simulink model "Hardware_Model"  (R2022b)
settings: Solver=ode5  StartTime=0.0  StopTime=365  RelTol=1e-3  EnableMultiTasking=on
undefined symbols (not defined in the file or in its folder): cf, conv, sf, uc, vf
libraries: arduinolib x9, simulink x5, dspsigops x1
settings Model: SimulationMode=external  ExtModeTrigDuration=2  Creator=gotta  LastModifiedBy=gotta
settings SolverCC: AutoInsertRateTranBlk=on
settings OptimizationCC: EnhancedBackFolding=on  PassReuseOutputArgsAs=Individual arguments  ZeroExternalMemoryAtStartup=off  ZeroInternalMemoryAtStartup=off  MaxStackSize=64  OptimizeBlockOrder=speed  DifferentSizesBufferReuse=on  OptimizationCustomize=off  EfficientTunableParamExpr=on
settings DebuggingCC: ParameterTunabilityLossMsg=error
settings HardwareCC: ProdBitPerPointer=32  ProdBitPerSizeT=32  ProdBitPerPtrDiffT=32  ProdLargestAtomicInteger=Long  ProdLargestAtomicFloat=Double  ProdWordSize=32  ProdHWDeviceType=ARM Compatible->ARM Cortex
settings SFSimCC: MATLABDynamicMemAlloc=off
settings RTWCC: Description=Embedded Coder  SystemTargetFile=ert.tlc  HardwareBoard=ESP32-WROOM(Arduino Compatible)  TemplateMakefile=ert_default_tmf  Toolchain=ESP32  BuildConfiguration=Faster Runs
settings CodeAppCC: ForceParamTrailComments=on  IgnoreCustomStorageClasses=off  OperatorAnnotations=on  SimulinkDataObjDesc=on  SFDataObjDesc=on  InsertBlockDesc=on
settings ERTTargetCC: SupportContinuousTime=on  SupportVariableSizeSignals=on  ExtMode=on  ExtModeTransport=3  ExtModeStaticAlloc=on  ExtModeAutomaticAllocSize=off  ExtModeStaticAllocSize=65536  ExtModeMexFile=ext_xcp  ExtModeMexArgs=0 3 921600  ExtModeIntrfLevel=Level2 - Open

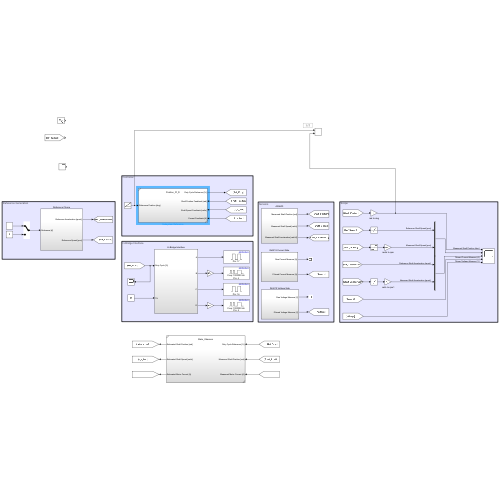
[thumbnail: Simulink's stored preview of the top-level diagram]
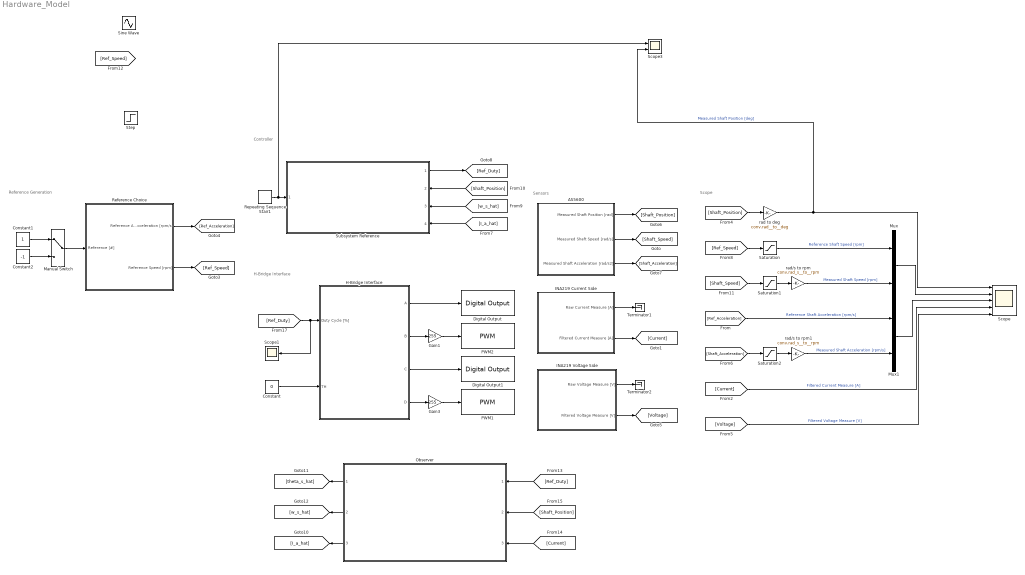
== system Hardware_Model ==
  note: Scope
  note: Sensors
  note: Controller
  note: H-Bridge Interface
  note: Reference Generation
  AS5600 : Subsystem
  Constant : Constant  Value=0
  Constant1 : Constant
  Constant2 : Constant  Value=-1
  Digital Output : arduinolib/Digital Output  pinNumber=17  Direction=output  blockPlatform=arduino
  Digital Output1 : arduinolib/Digital Output  pinNumber=16  Direction=output  blockPlatform=arduino
  Gain1 : Gain  Gain=255
  Gain3 : Gain  Gain=255
  H-Bridge Interface : Subsystem
  INA219 Current Side : Subsystem
  INA219 Voltage Side : Subsystem
  Manual Switch : ManualSwitch
  Mux : Mux  Inputs=2
  Mux1 : Mux  Inputs=2
  Observer : Subsystem  ReferencedSubsystem=State_Observer
  PWM1 : arduinolib/PWM  pinNumber=5  frequencyType=Specify  desiredFrequency=1e6  achievableFrequency=1000000
  PWM2 : arduinolib/PWM  pinNumber=4  frequencyType=Specify  desiredFrequency=1e6  achievableFrequency=1000000
  Reference Choice : Subsystem
  Repeating Sequence Stair1 : simulink/Sources/Repeating Sequence Stair  OutValues=5*[0:1:72]  tsamp=5  OutMin=[]  OutMax=[]  OutDataTypeStr=double  OutputDataTypeScalingMode=double  OutDataType=fixdt(0,8)  ConRadixGroup=Best Precision: Vector-wise  OutScaling=2^-12
  Saturation : Saturate  UpperLimit=130  LowerLimit=-130
  Saturation1 : Saturate  UpperLimit=130  LowerLimit=-130
  Saturation2 : Saturate  UpperLimit=50  LowerLimit=-50
  Scope : Scope  NumInputPorts=5
  Scope1 : Scope
  Scope3 : Scope  NumInputPorts=2
  Sine Wave : Sin  Amplitude=90  SampleTime=0
  Step : Step  After=100  SampleTime=0
  Subsystem Reference : Subsystem  ReferencedSubsystem=Position_PI_D
      settings: PortSchema="{\"entries\":[{\"content\":{\"sides\":[{\"content\":{\"connectorIds\":[\"In1\"]},\"type\":\"ConnectorPlacement.EquallySpacedRectSide\",\"uuid\":\"89c992bc-e0f3-428d-980e-b961eb5d7b7b\"},{\"content\":{\"connectorIds\":[\"Out1\",\"In2\",\"In3\",\"In4\"],\"side\":\"RIGHT\"},\"type\":\"ConnectorPlacement.EquallySpacedRectSide\",\"uuid\":\"dbaab0ea-2322-47c9-b2e4-ea83bc14c20f\"},{\"content\":{\"connectorIds\":[],\"side\":\"TOP\"},\"type\":\"ConnectorPlacement.EquallySpacedRectSide\",\"uuid\":\"a9d5f6a0-5f2c-4e6a-b514-fb4908ab5e4d\"}]},\"type\":\"ConnectorPlacement.EquallySpacedConnector\",\"uuid\":\"ac98b5ea-1932-4944-bc3f-916f19a2da62\"}],\"packageUris\":[\"http://schema.mathworks.com/mf0/Connector/R2020b\"],\"version\":\"1.0\"}"
  Terminator1 : Terminator
  Terminator2 : Terminator
  rad to deg : Gain  Gain=conv.rad__to__deg
  rad/s to rpm : Gain  Gain=conv.rad_s__to__rpm
  rad/s to rpm1 : Gain  Gain=conv.rad_s__to__rpm
  wires:
  Manual Switch/1 -> Reference Choice/1(Reference [#])
  Constant1/1 -> Manual Switch/1
  Constant2/1 -> Manual Switch/2
  Reference Choice/1(Reference Acceleration [rpm/s]) -> [Ref_Acceleration]
  Reference Choice/2(Reference Speed [rpm]) -> [Ref_Speed]
  H-Bridge Interface/4(D) -> Gain3/1
  H-Bridge Interface/2(B) -> Gain1/1
  H-Bridge Interface/3(C) -> Digital Output1/1
  [Ref_Duty] -> Scope1/1, H-Bridge Interface/1(Duty Cycle [%])
  Constant/1 -> H-Bridge Interface/2(TH)
  H-Bridge Interface/1(A) -> Digital Output/1
  Gain1/1 -> PWM2/1
  Gain3/1 -> PWM1/1
  INA219 Current Side/2(Filtered Current Measure [A]) -> [Current]
  AS5600/2(Measured Shaft Speed [rad/s]) -> [Shaft_Speed]
  INA219 Voltage Side/2(Filtered Voltage Measure [V]) -> [Voltage]
  AS5600/3(Measured Shaft Acceleration [rad/s2]) -> [Shaft_Acceleration]
  AS5600/1(Measured Shaft Position [rad]) -> [Shaft_Position]
  [Current] -> Scope/4  "Filtered Current Measure [A]"
  Saturation1/1 -> rad/s to rpm/1
  Saturation/1 -> Mux/1  "Reference Shaft Speed [rpm]"
  [Shaft_Acceleration] -> Saturation2/1
  Mux/1 -> Scope/2
  rad/s to rpm1/1 -> Mux1/2  "Measured Shaft Acceleration [rpm/s]"
  [Ref_Acceleration] -> Mux1/1  "Reference Shaft Acceleration [rpm/s]"
  rad/s to rpm/1 -> Mux/2  "Measured Shaft Speed [rpm]"
  [Shaft_Speed] -> Saturation1/1
  [Ref_Speed] -> Saturation/1
  [Voltage] -> Scope/5  "Filtered Voltage Measure [V]"
  [Shaft_Position] -> rad to deg/1
  Mux1/1 -> Scope/3
  rad to deg/1 -> Scope3/2, Scope/1  "Measured Shaft Position [deg]"
  Saturation2/1 -> rad/s to rpm1/1
  INA219 Current Side/1(Raw Current Measure [A]) -> Terminator1/1
  INA219 Voltage Side/1(Raw Voltage Measure [V]) -> Terminator2/1
  [I_a_hat] -> Subsystem Reference/4
  [w_s_hat] -> Subsystem Reference/3
  [Shaft_Position] -> Subsystem Reference/2
  Observer/1 -> [theta_s_hat]
  Observer/3 -> [I_a_hat]
  Observer/2 -> [w_s_hat]
  [Ref_Duty] -> Observer/1
  [Current] -> Observer/3
  [Shaft_Position] -> Observer/2
  Subsystem Reference/1 -> [Ref_Duty]
  Repeating Sequence Stair1/1 -> Scope3/1, Subsystem Reference/1

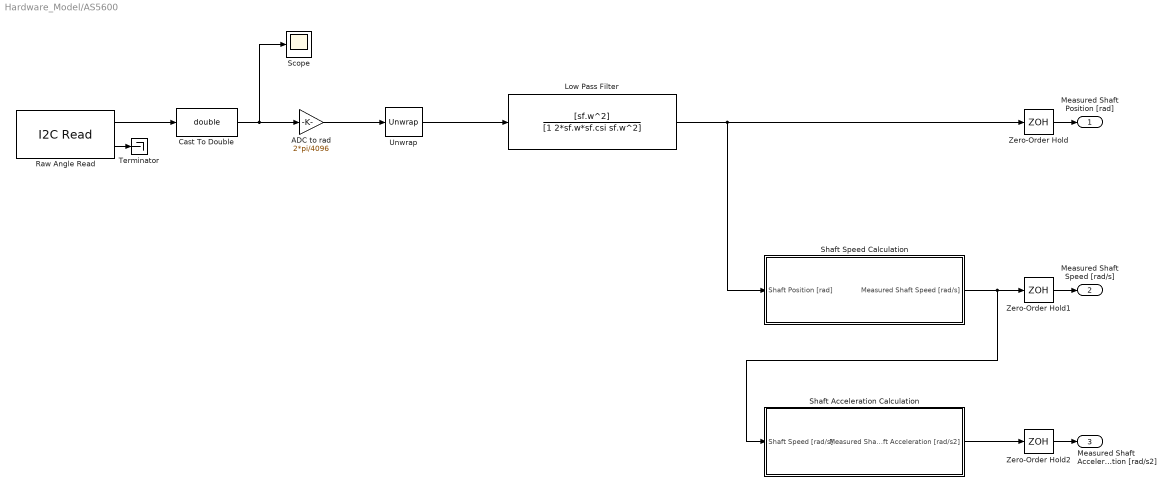
== system Hardware_Model/AS5600 ==
  ADC to rad : Gain  Gain=2*pi/4096
  Cast To Double : DataTypeConversion  OutDataTypeStr=double  SaturateOnIntegerOverflow=off  RndMeth=Floor
  Low Pass Filter : TransferFcn  Numerator=[sf.w^2]  Denominator=[1 2*sf.w*sf.csi sf.w^2]
  Raw Angle Read : arduinolib/I2C Read  I2CModule=0  Mode=Master  SlaveAddress=0x36  SlaveByteOrder=BigEndian  Direction=Receiver  RegisterAddressMode=on  RegisterAddress=0x0C  SlaveDataType=uint16  DataLength=1  NoAck=off  RepeatedStart=off  OutputStatus=on  blockPlatform=ARDUINO  SampleTime=uc.Ts
  Scope : Scope
  Shaft Acceleration Calculation : Subsystem
  Shaft Speed Calculation : Subsystem
  Terminator : Terminator
  Unwrap : dspsigops/Unwrap  tol=pi  InputProcessing=Columns as channels (frame based)  running=off
  Zero-Order Hold : ZeroOrderHold  SampleTime=uc.Ts
  Zero-Order Hold1 : ZeroOrderHold  SampleTime=uc.Ts
  Zero-Order Hold2 : ZeroOrderHold  SampleTime=uc.Ts
  Measured Shaft Position [rad] : Outport
  Measured Shaft Speed [rad/s] : Outport  Port=2
  Measured Shaft Acceleration [rad/s2] : Outport  Port=3
  wires:
  ADC to rad/1 -> Unwrap/1
  Cast To Double/1 -> Scope/1, ADC to rad/1
  Raw Angle Read/1 -> Cast To Double/1
  Unwrap/1 -> Low Pass Filter/1
  Raw Angle Read/2 -> Terminator/1
  Shaft Speed Calculation/1(Measured Shaft Speed [rad/s]) -> Shaft Acceleration Calculation/1(Shaft Speed [rad/s]), Zero-Order Hold1/1
  Shaft Acceleration Calculation/1(Measured Shaft Acceleration [rad/s2]) -> Zero-Order Hold2/1
  Low Pass Filter/1 -> Shaft Speed Calculation/1(Shaft Position [rad]), Zero-Order Hold/1
  Zero-Order Hold/1 -> Measured Shaft Position [rad]/1
  Zero-Order Hold1/1 -> Measured Shaft Speed [rad/s]/1
  Zero-Order Hold2/1 -> Measured Shaft Acceleration [rad/s2]/1

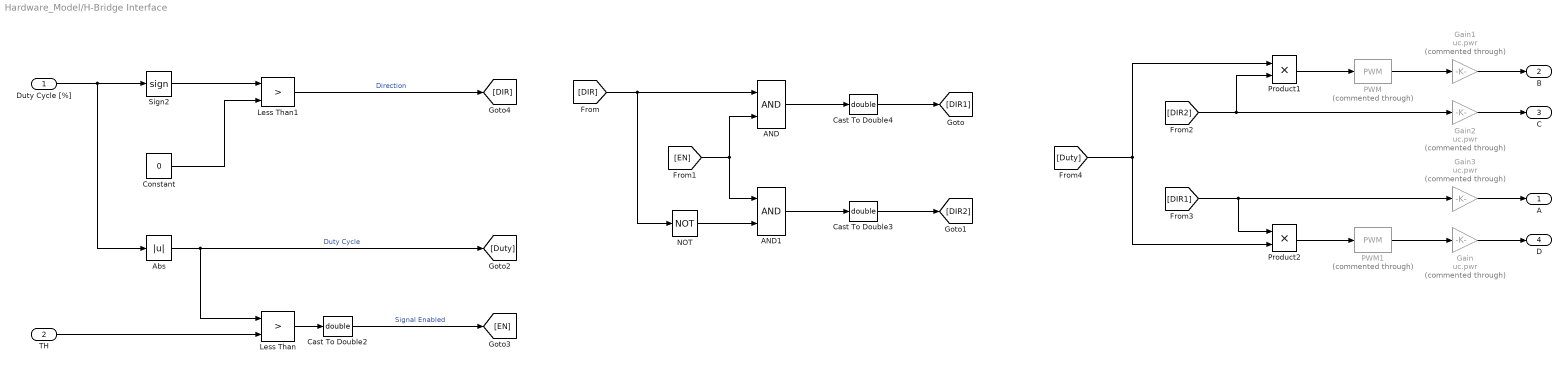
== system Hardware_Model/H-Bridge Interface ==
  Duty Cycle [%] : Inport
  TH : Inport  Port=2
  AND : Logic  IconShape=distinctive  AllPortsSameDT=off  OutDataTypeStr=boolean
  AND1 : Logic  IconShape=distinctive  AllPortsSameDT=off  OutDataTypeStr=boolean
  Abs : Abs  SaturateOnIntegerOverflow=off
  Cast To Double2 : DataTypeConversion  OutDataTypeStr=double  SaturateOnIntegerOverflow=off  RndMeth=Floor
  Cast To Double3 : DataTypeConversion  OutDataTypeStr=double  SaturateOnIntegerOverflow=off  RndMeth=Floor
  Cast To Double4 : DataTypeConversion  OutDataTypeStr=double  SaturateOnIntegerOverflow=off  RndMeth=Floor
  Constant : Constant  Value=0
  Gain{,1..3} (4 alike) : Gain  Commented=through  Gain=uc.pwr
  Less Than : RelationalOperator  Operator=>  OutDataTypeStr=boolean  RndMeth=Simplest  InputSameDT=off
  Less Than1 : RelationalOperator  Operator=>  OutDataTypeStr=boolean  RndMeth=Simplest  InputSameDT=off
  NOT : Logic  Operator=NOT  IconShape=distinctive  AllPortsSameDT=off  OutDataTypeStr=boolean
  PWM : simulink/Discontinuities/PWM  Commented=through  DisableCoverage=on  Period=uc.Tpwm  InitialDelay=0  DisallowZeroDutyCycle=off  RunAtFixedTimeIntervals=on  SampleTime=uc.Tpwm/10
  PWM1 : simulink/Discontinuities/PWM  Commented=through  DisableCoverage=on  Period=uc.Tpwm  InitialDelay=0  DisallowZeroDutyCycle=off  RunAtFixedTimeIntervals=on  SampleTime=uc.Tpwm/10
  Product1 : Product
  Product2 : Product
  Sign2 : Signum
  A : Outport
  B : Outport  Port=2
  C : Outport  Port=3
  D : Outport  Port=4
  wires:
  TH/1 -> Less Than/2
  Duty Cycle [%]/1 -> Abs/1, Sign2/1
  Less Than/1 -> Cast To Double2/1
  Sign2/1 -> Less Than1/1
  Constant/1 -> Less Than1/2
  Abs/1 -> [Duty], Less Than/1  "Duty Cycle"
  Gain/1 -> D/1
  Gain1/1 -> B/1
  Gain2/1 -> C/1
  Gain3/1 -> A/1
  AND1/1 -> Cast To Double3/1
  AND/1 -> Cast To Double4/1
  NOT/1 -> AND1/2
  Product1/1 -> PWM/1
  Product2/1 -> PWM1/1
  Cast To Double2/1 -> [EN]  "Signal Enabled"
  Less Than1/1 -> [DIR]  "Direction"
  [DIR] -> NOT/1, AND/1
  [EN] -> AND/2, AND1/1
  Cast To Double4/1 -> [DIR1]
  Cast To Double3/1 -> [DIR2]
  [DIR2] -> Product1/2, Gain2/1
  [DIR1] -> Product2/1, Gain3/1
  [Duty] -> Product1/1, Product2/2
  PWM/1 -> Gain1/1
  PWM1/1 -> Gain/1

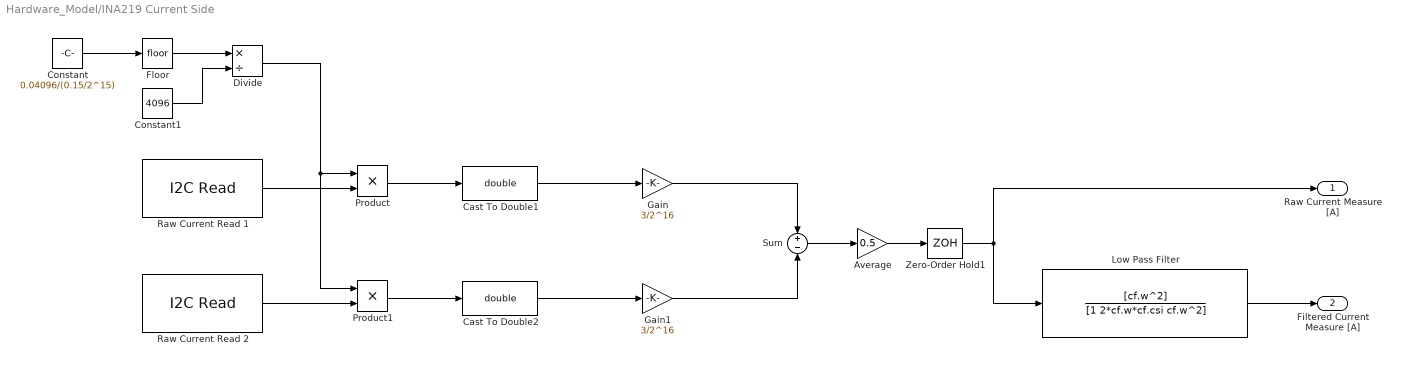
== system Hardware_Model/INA219 Current Side ==
  Average : Gain  Gain=0.5
  Cast To Double1 : DataTypeConversion  OutDataTypeStr=double  SaturateOnIntegerOverflow=off  RndMeth=Floor
  Cast To Double2 : DataTypeConversion  OutDataTypeStr=double  SaturateOnIntegerOverflow=off  RndMeth=Floor
  Constant : Constant  Value=0.04096/(0.15/2^15)
  Constant1 : Constant  Value=4096
  Divide : Product  Inputs=*/
  Floor : Rounding
  Gain : Gain  Gain=3/2^16
  Gain1 : Gain  Gain=3/2^16
  Low Pass Filter : TransferFcn  Numerator=[cf.w^2]  Denominator=[1 2*cf.w*cf.csi cf.w^2]
  Product : Product
  Product1 : Product
  Raw Current Read 1 : arduinolib/I2C Read  I2CModule=0  Mode=Master  SlaveAddress=0x40  SlaveByteOrder=BigEndian  Direction=Receiver  RegisterAddressMode=on  RegisterAddress=0x01  SlaveDataType=int16  DataLength=1  NoAck=off  RepeatedStart=off  OutputStatus=off  blockPlatform=ARDUINO  SampleTime=uc.Ts
  Raw Current Read 2 : arduinolib/I2C Read  I2CModule=0  Mode=Master  SlaveAddress=0x44  SlaveByteOrder=BigEndian  Direction=Receiver  RegisterAddressMode=on  RegisterAddress=0x01  SlaveDataType=int16  DataLength=1  NoAck=off  RepeatedStart=off  OutputStatus=off  blockPlatform=ARDUINO  SampleTime=uc.Ts
  Sum : Sum  Inputs=+|-
  Zero-Order Hold1 : ZeroOrderHold  SampleTime=uc.Ts
  Raw Current Measure [A] : Outport
  Filtered Current Measure [A] : Outport  Port=2
  wires:
  Average/1 -> Zero-Order Hold1/1
  Sum/1 -> Average/1
  Low Pass Filter/1 -> Filtered Current Measure [A]/1
  Constant/1 -> Floor/1
  Floor/1 -> Divide/1
  Constant1/1 -> Divide/2
  Raw Current Read 2/1 -> Product1/2
  Raw Current Read 1/1 -> Product/2
  Divide/1 -> Product1/1, Product/1
  Product/1 -> Cast To Double1/1
  Product1/1 -> Cast To Double2/1
  Gain/1 -> Sum/1
  Gain1/1 -> Sum/2
  Cast To Double1/1 -> Gain/1
  Cast To Double2/1 -> Gain1/1
  Zero-Order Hold1/1 -> Low Pass Filter/1, Raw Current Measure [A]/1

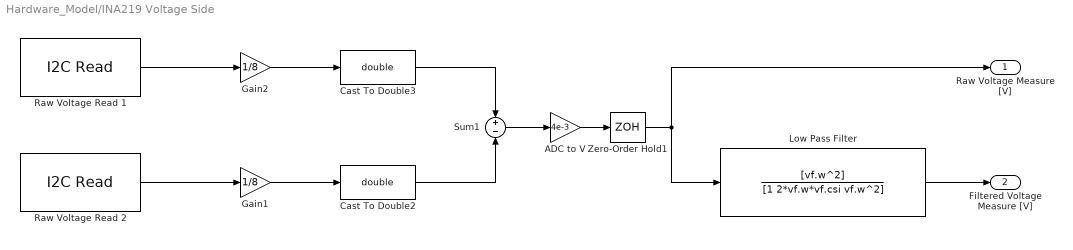
== system Hardware_Model/INA219 Voltage Side ==
  ADC to V : Gain  Gain=4e-3
  Cast To Double2 : DataTypeConversion  OutDataTypeStr=double  SaturateOnIntegerOverflow=off  RndMeth=Floor
  Cast To Double3 : DataTypeConversion  OutDataTypeStr=double  SaturateOnIntegerOverflow=off  RndMeth=Floor
  Gain1 : Gain  Gain=1/8
  Gain2 : Gain  Gain=1/8
  Low Pass Filter : TransferFcn  Numerator=[vf.w^2]  Denominator=[1 2*vf.w*vf.csi vf.w^2]
  Raw Voltage Read 1 : arduinolib/I2C Read  I2CModule=0  Mode=Master  SlaveAddress=0x40  SlaveByteOrder=BigEndian  Direction=Receiver  RegisterAddressMode=on  RegisterAddress=0x02  SlaveDataType=uint16  DataLength=1  NoAck=off  RepeatedStart=off  OutputStatus=off  blockPlatform=ARDUINO  SampleTime=uc.Ts
  Raw Voltage Read 2 : arduinolib/I2C Read  I2CModule=0  Mode=Master  SlaveAddress=0x44  SlaveByteOrder=BigEndian  Direction=Receiver  RegisterAddressMode=on  RegisterAddress=0x02  SlaveDataType=uint16  DataLength=1  NoAck=off  RepeatedStart=off  OutputStatus=off  blockPlatform=ARDUINO  SampleTime=uc.Ts
  Sum1 : Sum  Inputs=+|-
  Zero-Order Hold1 : ZeroOrderHold  SampleTime=uc.Ts
  Raw Voltage Measure [V] : Outport
  Filtered Voltage Measure [V] : Outport  Port=2
  wires:
  Cast To Double2/1 -> Sum1/2
  Gain1/1 -> Cast To Double2/1
  Raw Voltage Read 1/1 -> Gain2/1
  Sum1/1 -> ADC to V/1
  Raw Voltage Read 2/1 -> Gain1/1
  Gain2/1 -> Cast To Double3/1
  Cast To Double3/1 -> Sum1/1
  ADC to V/1 -> Zero-Order Hold1/1
  Low Pass Filter/1 -> Filtered Voltage Measure [V]/1
  Zero-Order Hold1/1 -> Low Pass Filter/1, Raw Voltage Measure [V]/1

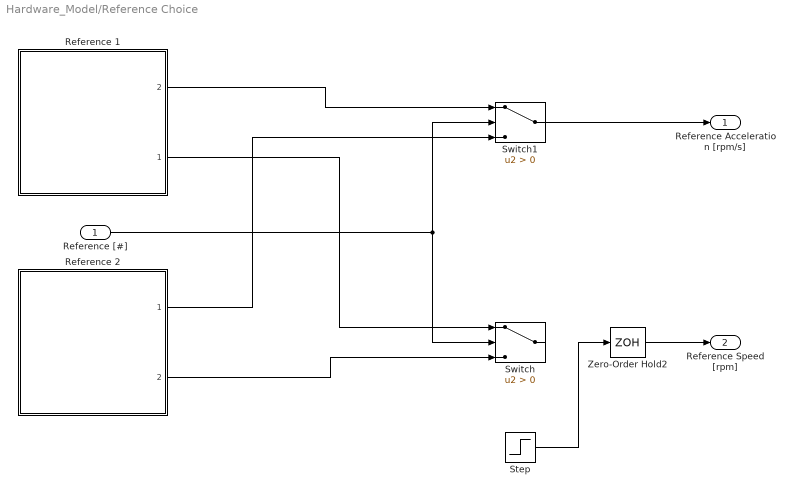
== system Hardware_Model/Reference Choice ==
  Reference [#] : Inport
  Reference 1 : Subsystem  ReferencedSubsystem=Staircase_Speed
      settings: PortSchema="{\"entries\":[{\"content\":{\"sides\":[{\"content\":{\"connectorIds\":[]},\"type\":\"ConnectorPlacement.EquallySpacedRectSide\",\"uuid\":\"9885add8-8968-49eb-949f-a37df14b92b0\"},{\"content\":{\"connectorIds\":[\"Out2\",\"Out1\"],\"side\":\"RIGHT\"},\"type\":\"ConnectorPlacement.EquallySpacedRectSide\",\"uuid\":\"3161d467-5fd0-4a02-8f79-2d64402fae8e\"},{\"content\":{\"connectorIds\":[],\"side\":\"TOP\"},\"type\":\"ConnectorPlacement.EquallySpacedRectSide\",\"uuid\":\"6f44884f-fb08-4fcd-b91b-4054e141836e\"}]},\"type\":\"ConnectorPlacement.EquallySpacedConnector\",\"uuid\":\"138f5dae-bb02-4292-8945-548fe1101b6c\"}],\"packageUris\":[\"http://schema.mathworks.com/mf0/Connector/R2020b\"],\"version\":\"1.0\"}"
  Reference 2 : Subsystem  ReferencedSubsystem=Triangle_Speed
  Step : Step  After=100  SampleTime=0
  Switch : Switch  Criteria=u2 > Threshold  SaturateOnIntegerOverflow=off  InputSameDT=off
  Switch1 : Switch  Criteria=u2 > Threshold  SaturateOnIntegerOverflow=off  InputSameDT=off
  Zero-Order Hold2 : ZeroOrderHold  SampleTime=uc.Ts
  Reference Acceleration [rpm/s] : Outport
  Reference Speed [rpm] : Outport  Port=2
  wires:
  Reference 1/2 -> Switch1/1
  Reference 1/1 -> Switch/1
  Reference [#]/1 -> Switch/2, Switch1/2
  Switch1/1 -> Reference Acceleration [rpm/s]/1
  Zero-Order Hold2/1 -> Reference Speed [rpm]/1
  Reference 2/2 -> Switch/3
  Reference 2/1 -> Switch1/3
  Step/1 -> Zero-Order Hold2/1

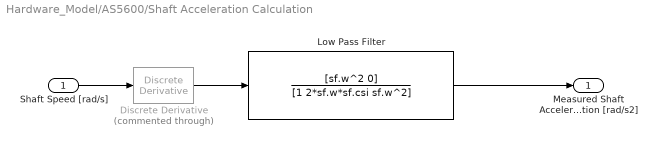
== system Hardware_Model/AS5600/Shaft Acceleration Calculation ==
  Shaft Speed [rad/s] : Inport
  Discrete Derivative : simulink/Discrete/Discrete Derivative  Commented=through  gainval=1.0  ICPrevScaledInput=0.0  OutMin=[]  OutMax=[]  OutDataType=fixdt(1, 16)  OutScaling=2^-10  DoSatur=off
  Low Pass Filter : TransferFcn  Numerator=[sf.w^2 0]  Denominator=[1 2*sf.w*sf.csi sf.w^2]
  Measured Shaft Acceleration [rad/s2] : Outport
  wires:
  Low Pass Filter/1 -> Measured Shaft Acceleration [rad/s2]/1
  Shaft Speed [rad/s]/1 -> Discrete Derivative/1
  Discrete Derivative/1 -> Low Pass Filter/1

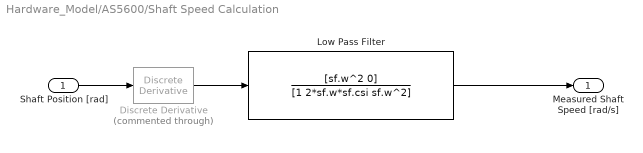
== system Hardware_Model/AS5600/Shaft Speed Calculation ==
  Shaft Position [rad] : Inport
  Discrete Derivative : simulink/Discrete/Discrete Derivative  Commented=through  gainval=1.0  ICPrevScaledInput=0.0  OutMin=[]  OutMax=[]  OutDataType=fixdt(1, 16)  OutScaling=2^-10  DoSatur=off
  Low Pass Filter : TransferFcn  Numerator=[sf.w^2 0]  Denominator=[1 2*sf.w*sf.csi sf.w^2]
  Measured Shaft Speed [rad/s] : Outport
  wires:
  Discrete Derivative/1 -> Low Pass Filter/1
  Shaft Position [rad]/1 -> Discrete Derivative/1
  Low Pass Filter/1 -> Measured Shaft Speed [rad/s]/1
